simulink model "regulacja"  (R2013a)
settings: Solver=ode45  SolverMode=SingleTasking  StartTime=0.0  StopTime=10.0  MaxStep=maxstepsize  RelTol=1e-3
values from neighbouring files (symbols this model uses):
  dTwew1_0 = 2    [identyfikacja transmitancji.m]    (also in skrypt.m)
  ki = kp/Ti    (= 4.52196844658e-06)    [identyfikacja transmitancji.m]    (also in skrypt.m = kp/Ti)
  kp = 0.9 * T3 /(k3*T30)    (= 0.173168781662)    [identyfikacja transmitancji.m]    (also in skrypt.m = 0.65*kp)
  L = [k3]    [identyfikacja transmitancji.m]
  M = [T3 ,1]    [identyfikacja transmitancji.m]
  steptime = czas*10^(-2)    (= 10000)    [skrypt.m]
  T30 = 11500    [identyfikacja transmitancji.m]
  Twew1_0 = (Kcg1*C_1*(Kcw1+Kcs1)*Tgz1_0+Kcw1*Kcs1*(Kcg1+C_1)*Tzew0)/M_1    (= 20)    [skrypt.m]
settings Model: Creator=r3vus  LastModifiedBy=LAB320-1552
settings DataIOCC: SignalLoggingSaveFormat=ModelDataLogs
settings OptimizationCC: BlockReduction=off  BooleanDataType=off
settings DebuggingCC: SaveWithParameterizedLinksMsg=none  SignalResolutionControl=TryResolveAllWithWarning  SolverPrmCheckMsg=none  MultiTaskDSMMsg=warning  MultiTaskCondExecSysMsg=none  StrictBusMsg=None
settings HardwareCC: TargetUnknown=on
settings RTWCC: IncludeERTFirstTime=on

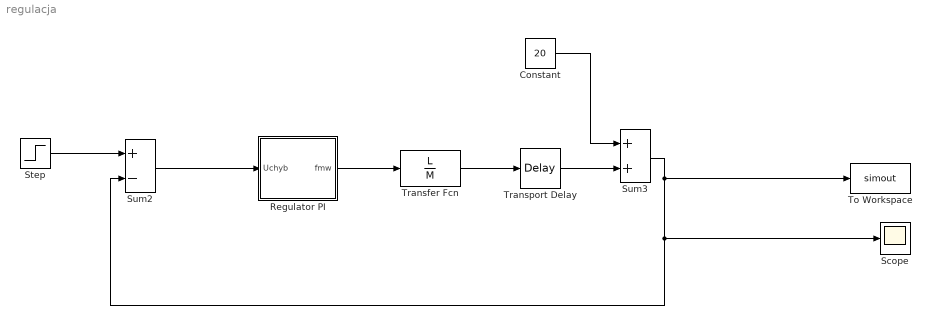
== system regulacja ==
  Constant : Constant  Value=20
  Regulator PI : Subsystem
  Scope : Scope
  Step : Step  Time=steptime  Before=Twew1_0  After=Twew1_0+dTwew1_0  SampleTime=0  VectorParams1D=off
  Sum2 : Sum  Inputs=+-
  Sum3 : Sum
  To Workspace : ToWorkspace  VariableName=simout  SampleTime=-1
  Transfer Fcn : TransferFcn  Numerator=L  Denominator=M
  Transport Delay : TransportDelay  DelayTime=T30
  wires:
  Step/1 -> Sum2/1
  Transfer Fcn/1 -> Transport Delay/1
  Transport Delay/1 -> Sum3/2
  Sum3/1 -> To Workspace/1, Scope/1, Sum2/2
  Constant/1 -> Sum3/1
  Sum2/1 -> Regulator PI/1(Uchyb)
  Regulator PI/1(fmw) -> Transfer Fcn/1

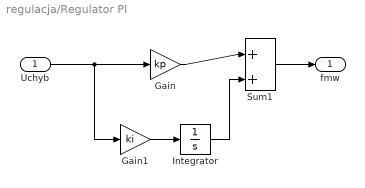
== system regulacja/Regulator PI ==
  Uchyb : Inport
  Gain : Gain  Gain=kp
  Gain1 : Gain  Gain=ki
  Integrator : Integrator
  Sum1 : Sum  Inputs=|++
  fmw : Outport
  wires:
  Sum1/1 -> fmw/1
  Integrator/1 -> Sum1/2
  Gain1/1 -> Integrator/1
  Uchyb/1 -> Gain1/1, Gain/1
  Gain/1 -> Sum1/1
